simulink model "StateMessage"  (R2024a)
settings: Solver=FixedStepAuto  StartTime=0.0  StopTime=0  FixedStep=0.01  RelTol=1e-3  EnableMultiTasking=on
libraries: MESSIN_Library x3
settings Model: Creator=damerius  LastModifiedBy=Scythe
settings SolverCC: ConcurrentTasks=on  AlgebraicLoopSolver=TrustRegion  PositivePriorityOrder=on
settings DataIOCC: SaveOutput=off  SignalLogging=off  DSMLogging=off  SaveTime=off  ReturnWorkspaceOutputs=off
settings OptimizationCC: DefaultParameterBehavior=Inlined  ReuseModelBlockBuffer=off  ZeroExternalMemoryAtStartup=off  ZeroInternalMemoryAtStartup=off  SimCompilerOptimization=on
settings DebuggingCC: UnconnectedInputMsg=warning  UnconnectedOutputMsg=warning  UnconnectedLineMsg=warning
settings HardwareCC: ProdBitPerLong=64  ProdHWDeviceType=Intel->x86-64 (Linux 64)
settings ModelReferenceCC: EnableRefExpFcnMdlSchedulingChecks=on
settings SFSimCC: SimParseCustomCode=off  SimGenImportedTypeDefs=on  SimTargetLang=C++
settings RTWCC: GenCodeOnly=on  PackageGeneratedCodeAndArtifacts=on  PackageName=PackNGo  RTWVerbose=off  BuildConfiguration=Faster Runs  TargetLang=C++  GPUComputeCapability=3.5  DLArmComputeVersion=19.05
settings CodeAppCC: ForceParamTrailComments=on  MaxIdLength=95  MATLABSourceComments=on  UseSimReservedNames=on
settings GRTTargetCC: TargetLangStandard=C++11 (ISO)  GenerateFullHeader=off  MatFileLogging=off  CodeInterfacePackaging=C++ class

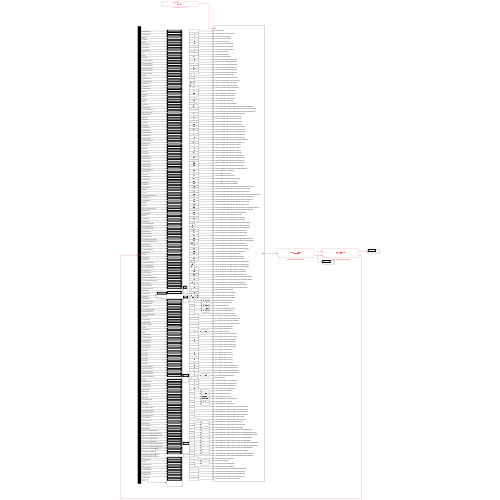
[thumbnail: Simulink's stored preview of the top-level diagram]
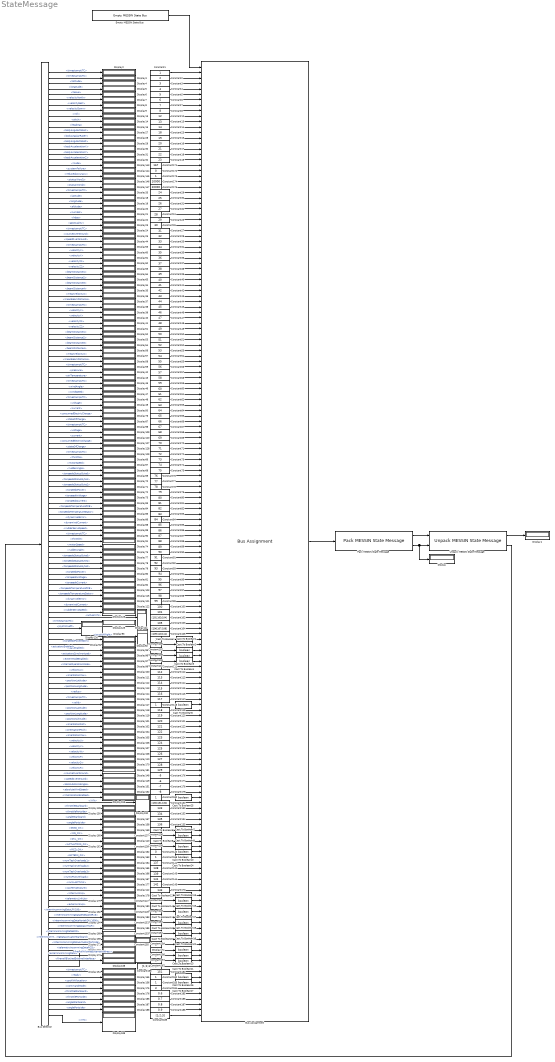
== system StateMessage ==
  Bus Assignment : BusAssignment  AssignedSignals=timestampUTC,sensor.insLFK100.timestampUTC,sensor.insLFK100.latitude,sensor.insLFK100.longitude,sensor.insLFK100.heave,sensor.insLFK100.velocityNorth,sensor.insLFK100.velocityEast,sensor.insLFK100.velocityDown,sensor.insLFK100.roll,sensor.insLFK100.pitch,sensor.insLFK100.heading,sensor.insLFK100.bodyAngularRateX,sensor.insLFK100.bodyAngularRateY,sensor.insLFK100.bodyAngularRateZ,sensor.insLFK100.bodyAccelerationX,sensor.insLFK100.bodyAccelerationY,sensor.insLFK100.bodyAccelerationZ,sensor.insLFK100.details.mode,sensor.insLFK100.details.systemFailure,sensor.insLFK100.details.reducedAccuracy,sensor.insLFK100.details.statusWord1,sensor.insLFK100.details.statusWord2,sensor.gnssAsteRx3.gnss.timestampUTC,sensor.gnssAsteRx3.gnss.latitude,sensor.gnssAsteRx3.gnss.longitude,sensor.gnssAsteRx3.gnss.altitude,sensor.gnssAsteRx3.gnss.numSat,sensor.gnssAsteRx3.gnss.hdop,sensor.gnssAsteRx3.gnss.gpsQuality,sensor.gnssAsteRx3.courseAndSpeedOverGround.timestampUTC,sensor.gnssAsteRx3.courseAndSpeedOverGround.courseOverGround,sensor.gnssAsteRx3.courseAndSpeedOverGround.speedOverGround,sensor.nortekDVL1000.bottomTrack.timestampUTC,sensor.nortekDVL1000.bottomTrack.velocityX,sensor.nortekDVL1000.bottomTrack.velocityY,sensor.nortekDVL1000.bottomTrack.velocityZ1,sensor.nortekDVL1000.bottomTrack.velocityZ2,sensor.nortekDVL1000.bottomTrack.beamDistance1,sensor.nortekDVL1000.bottomTrack.beamDistance2,sensor.nortekDVL1000.bottomTrack.beamDistance3,sensor.nortekDVL1000.bottomTrack.beamDistance4,sensor.nortekDVL1000.bottomTrack.meanVelocityZ,sensor.nortekDVL1000.bottomTrack.meanBeamDistance,sensor.nortekDVL1000.waterTrack.timestampUTC,sensor.nortekDVL1000.waterTrack.velocityX,sensor.nortekDVL1000.waterTrack.velocityY,sensor.nortekDVL1000.waterTrack.velocityZ1,sensor.nortekDVL1000.waterTrack.velocityZ2,sensor.nortekDVL1000.waterTrack.beamDistance1,sensor.nortekDVL1000.waterTrack.beamDistance2,sensor.nortekDVL1000.waterTrack.beamDistance3,sensor.nortekDVL1000.waterTrack.beamDistance4,sensor.nortekDVL1000.waterTrack.meanVelocityZ,sensor.nortekDVL1000.waterTrack.meanBeamDistance,sensor.airMAR.air.timestampUTC,sensor.airMAR.air.pressure,sensor.airMAR.air.airTemperature,sensor.airMAR.relativeWind.timestampUTC,sensor.airMAR.relativeWind.windAngle,sensor.airMAR.relativeWind.windSpeed,sensor.batteryManagementSystem.batteryStarboard.timestampUTC,sensor.batteryManagementSystem.batteryStarboard.voltage,sensor.batteryManagementSystem.batteryStarboard.current,sensor.batteryManagementSystem.batteryStarboard.consumedElectricCharge,sensor.batteryManagementSystem.batteryStarboard.stateOfCharge,sensor.batteryManagementSystem.batteryPortside.timestampUTC,sensor.batteryManagementSystem.batteryPortside.voltage,sensor.batteryManagementSystem.batteryPortside.current,sensor.batteryManagementSystem.batteryPortside.consumedElectricCharge,sensor.batteryManagementSystem.batteryPortside.stateOfCharge,sensor.messinDrive.actuatorStarboard.timestampUTC,sensor.messinDrive.actuatorStarboard.throttle,sensor.messinDrive.actuatorStarboard.motorSpeed,sensor.messinDrive.actuatorStarboard.rudderAngle,sensor.messinDrive.actuatorStarboard.torqeedoStatusByte0,sensor.messinDrive.actuatorStarboard.torqeedoStatusByte1,sensor.messinDrive.actuatorStarboard.torqeedoStatusByte2,sensor.messinDrive.actuatorStarboard.torqeedoPower,sensor.messinDrive.actuatorStarboard.torqeedoVoltage,sensor.messinDrive.actuatorStarboard.torqeedoCurrent,sensor.messinDrive.actuatorStarboard.torqeedoTemperaturePCB,sensor.messinDrive.actuatorStarboard.torqeedoTemperatureStator,sensor.messinDrive.actuatorStarboard.dynamixelError,sensor.messinDrive.actuatorStarboard.dynamixelCurrent,sensor.messinDrive.actuatorStarboard.rudderServoSpeed,sensor.messinDrive.actuatorPortside.timestampUTC,sensor.messinDrive.actuatorPortside.throttle,sensor.messinDrive.actuatorPortside.motorSpeed,sensor.messinDrive.actuatorPortside.rudderAngle,sensor.messinDrive.actuatorPortside.torqeedoStatusByte0,sensor.messinDrive.actuatorPortside.torqeedoStatusByte1,sensor.messinDrive.actuatorPortside.torqeedoStatusByte2,sensor.messinDrive.actuatorPortside.torqeedoPower,sensor.messinDrive.actuatorPortside.torqeedoVoltage,sensor.messinDrive.actuatorPortside.torqeedoCurrent,sensor.messinDrive.actuatorPortside.torqeedoTemperaturePCB,sensor.messinDrive.actuatorPortside.torqeedoTemperatureStator,sensor.messinDrive.actuatorPortside.dynamixelError,sensor.messinDrive.actuatorPortside.dynamixelCurrent,sensor.messinDrive.actuatorPortside.rudderServoSpeed,sensor.messinDrive.actualXYN,remoteControlDevice.timestampUTC,remoteControlDevice.joystickLeft,remoteControlDevice.joystickRight,supervisor.torqeedoPoweredOn,supervisor.actuatorsEnabled,supervisor.lightEnabled,supervisor.actuatorsSynchronized,supervisor.externModeEnabled,supervisor.internalOperationMode,gnc.guidance.surgeHeading.velocityU,gnc.guidance.surgeHeading.orientationYaw,gnc.guidance.stayThere.positionLatitude,gnc.guidance.stayThere.positionLongitude,gnc.guidance.stayThere.radius,gnc.navigation.timestampUTC,gnc.navigation.info.valid,gnc.navigation.state.positionLatitude,gnc.navigation.state.positionLongitude,gnc.navigation.state.positionAltitude,gnc.navigation.state.orientationRoll,gnc.navigation.state.orientationPitch,gnc.navigation.state.orientationYaw,gnc.navigation.state.velocityU,gnc.navigation.state.velocityV,gnc.navigation.state.velocityW,gnc.navigation.state.velocityP,gnc.navigation.state.velocityQ,gnc.navigation.state.velocityR,gnc.navigation.state.courseOverGround,gnc.navigation.state.speedOverGround,gnc.navigation.state.absoluteWindAngle,gnc.navigation.state.absoluteWindSpeed,gnc.control.XNAllocationEnabled,gnc.control.XYN,commandedActuator.throttleStarboard,commandedActuator.throttlePortside,commandedActuator.angleStarboard,commandedActuator.anglePortside,systemDiagnostics.GNSS_OK,systemDiagnostics.INS_OK,systemDiagnostics.DVL_OK,systemDiagnostics.ACTUATORS_OK,systemDiagnostics.RCD_OK,systemDiagnostics.EXTERN_OK,systemDiagnostics.details.hardware.numTaskOverloads1,systemDiagnostics.details.hardware.numTaskOverloads2,systemDiagnostics.details.hardware.numTaskOverloads3,systemDiagnostics.details.hardware.numCPUOverloads,systemDiagnostics.details.hardware.numLostTicks,systemDiagnostics.details.hardware.cpuTemperature,systemDiagnostics.details.network.internLinkUp,systemDiagnostics.details.network.telemetryLinkUp,systemDiagnostics.details.network.externLinkUp,systemDiagnostics.details.network.internIncommingDataLFK100,systemDiagnostics.details.network.internIncommingDataGNSSAsteRx3,systemDiagnostics.details.network.internIncommingDataNortekDVL1000,systemDiagnostics.details.network.internIncommingDataAirMAR,systemDiagnostics.details.network.internIncommingDataBMS,systemDiagnostics.details.network.internIncommingDataActuatorStarboard,systemDiagnostics.details.network.internIncommingDataActuatorPortside,systemDiagnostics.details.network.telemetryIncommingDataRCD,systemDiagnostics.details.network.externIncommingData,systemDiagnostics.details.network.firewallBlockedExternalInterface,systemDiagnostics.details.network.firewallAllowedExternalAddress,externCommand.timestampUTC,externCommand.ready,externCommand.useXNAllocation,externCommand.commandMode,externCommand.actuatorCommand.throttleStarboard,externCommand.actuatorCommand.throttlePortside,externCommand.actuatorCommand.angleStarboard,externCommand.actuatorCommand.anglePortside,externCommand.allocationCommand.XYN
  Bus Selector : BusSelector  OutputSignals=timestampUTC,sensor.insLFK100.timestampUTC,sensor.insLFK100.latitude,sensor.insLFK100.longitude,sensor.insLFK100.heave,sensor.insLFK100.velocityNorth,sensor.insLFK100.velocityEast,sensor.insLFK100.velocityDown,sensor.insLFK100.roll,sensor.insLFK100.pitch,sensor.insLFK100.heading,sensor.insLFK100.bodyAngularRateX,sensor.insLFK100.bodyAngularRateY,sensor.insLFK100.bodyAngularRateZ,sensor.insLFK100.bodyAccelerationX,sensor.insLFK100.bodyAccelerationY,sensor.insLFK100.bodyAccelerationZ,sensor.insLFK100.details.mode,sensor.insLFK100.details.systemFailure,sensor.insLFK100.details.reducedAccuracy,sensor.insLFK100.details.statusWord1,sensor.insLFK100.details.statusWord2,sensor.gnssAsteRx3.gnss.timestampUTC,sensor.gnssAsteRx3.gnss.latitude,sensor.gnssAsteRx3.gnss.longitude,sensor.gnssAsteRx3.gnss.altitude,sensor.gnssAsteRx3.gnss.numSat,sensor.gnssAsteRx3.gnss.hdop,sensor.gnssAsteRx3.gnss.gpsQuality,sensor.gnssAsteRx3.courseAndSpeedOverGround.timestampUTC,sensor.gnssAsteRx3.courseAndSpeedOverGround.courseOverGround,sensor.gnssAsteRx3.courseAndSpeedOverGround.speedOverGround,sensor.nortekDVL1000.bottomTrack.timestampUTC,sensor.nortekDVL1000.bottomTrack.velocityX,sensor.nortekDVL1000.bottomTrack.velocityY,sensor.nortekDVL1000.bottomTrack.velocityZ1,sensor.nortekDVL1000.bottomTrack.velocityZ2,sensor.nortekDVL1000.bottomTrack.beamDistance1,sensor.nortekDVL1000.bottomTrack.beamDistance2,sensor.nortekDVL1000.bottomTrack.beamDistance3,sensor.nortekDVL1000.bottomTrack.beamDistance4,sensor.nortekDVL1000.bottomTrack.meanVelocityZ,sensor.nortekDVL1000.bottomTrack.meanBeamDistance,sensor.nortekDVL1000.waterTrack.timestampUTC,sensor.nortekDVL1000.waterTrack.velocityX,sensor.nortekDVL1000.waterTrack.velocityY,sensor.nortekDVL1000.waterTrack.velocityZ1,sensor.nortekDVL1000.waterTrack.velocityZ2,sensor.nortekDVL1000.waterTrack.beamDistance1,sensor.nortekDVL1000.waterTrack.beamDistance2,sensor.nortekDVL1000.waterTrack.beamDistance3,sensor.nortekDVL1000.waterTrack.beamDistance4,sensor.nortekDVL1000.waterTrack.meanVelocityZ,sensor.nortekDVL1000.waterTrack.meanBeamDistance,sensor.airMAR.air.timestampUTC,sensor.airMAR.air.pressure,sensor.airMAR.air.airTemperature,sensor.airMAR.relativeWind.timestampUTC,sensor.airMAR.relativeWind.windAngle,sensor.airMAR.relativeWind.windSpeed,sensor.batteryManagementSystem.batteryStarboard.timestampUTC,sensor.batteryManagementSystem.batteryStarboard.voltage,sensor.batteryManagementSystem.batteryStarboard.current,sensor.batteryManagementSystem.batteryStarboard.consumedElectricCharge,sensor.batteryManagementSystem.batteryStarboard.stateOfCharge,sensor.batteryManagementSystem.batteryPortside.timestampUTC,sensor.batteryManagementSystem.batteryPortside.voltage,sensor.batteryManagementSystem.batteryPortside.current,sensor.batteryManagementSystem.batteryPortside.consumedElectricCharge,sensor.batteryManagementSystem.batteryPortside.stateOfCharge,sensor.messinDrive.actuatorStarboard.timestampUTC,sensor.messinDrive.actuatorStarboard.throttle,sensor.messinDrive.actuatorStarboard.motorSpeed,sensor.messinDrive.actuatorStarboard.rudderAngle,sensor.messinDrive.actuatorStarboard.torqeedoStatusByte0,sensor.messinDrive.actuatorStarboard.torqeedoStatusByte1,sensor.messinDrive.actuatorStarboard.torqeedoStatusByte2,sensor.messinDrive.actuatorStarboard.torqeedoPower,sensor.messinDrive.actuatorStarboard.torqeedoVoltage,sensor.messinDrive.actuatorStarboard.torqeedoCurrent,sensor.messinDrive.actuatorStarboard.torqeedoTemperaturePCB,sensor.messinDrive.actuatorStarboard.torqeedoTemperatureStator,sensor.messinDrive.actuatorStarboard.dynamixelError,sensor.messinDrive.actuatorStarboard.dynamixelCurrent,sensor.messinDrive.actuatorStarboard.rudderServoSpeed,sensor.messinDrive.actuatorPortside.timestampUTC,sensor.messinDrive.actuatorPortside.throttle,sensor.messinDrive.actuatorPortside.motorSpeed,sensor.messinDrive.actuatorPortside.rudderAngle,sensor.messinDrive.actuatorPortside.torqeedoStatusByte0,sensor.messinDrive.actuatorPortside.torqeedoStatusByte1,sensor.messinDrive.actuatorPortside.torqeedoStatusByte2,sensor.messinDrive.actuatorPortside.torqeedoPower,sensor.messinDrive.actuatorPortside.torqeedoVoltage,sensor.messinDrive.actuatorPortside.torqeedoCurrent,sensor.messinDrive.actuatorPortside.torqeedoTemperaturePCB,sensor.messinDrive.actuatorPortside.torqeedoTemperatureStator,sensor.messinDrive.actuatorPortside.dynamixelError,sensor.messinDrive.actuatorPortside.dynamixelCurrent,sensor.messinDrive.actuatorPortside.rudderServoSpeed,sensor.messinDrive.actualXYN,remoteControlDevice.timestampUTC,remoteControlDevice.joystickLeft,remoteControlDevice.joystickRight,supervisor.torqeedoPoweredOn,supervisor.actuatorsEnabled,supervisor.lightEnabled,supervisor.actuatorsSynchronized,supervisor.externModeEnabled,supervisor.internalOperationMode,gnc.guidance.surgeHeading.velocityU,gnc.guidance.surgeHeading.orientationYaw,gnc.guidance.stayThere.positionLatitude,gnc.guidance.stayThere.positionLongitude,gnc.guidance.stayThere.radius,gnc.navigation.timestampUTC,gnc.navigation.info.valid,gnc.navigation.state.positionLatitude,gnc.navigation.state.positionLongitude,gnc.navigation.state.positionAltitude,gnc.navigation.state.orientationRoll,gnc.navigation.state.orientationPitch,gnc.navigation.state.orientationYaw,gnc.navigation.state.velocityU,gnc.navigation.state.velocityV,gnc.navigation.state.velocityW,gnc.navigation.state.velocityP,gnc.navigation.state.velocityQ,gnc.navigation.state.velocityR,gnc.navigation.state.courseOverGround,gnc.navigation.state.speedOverGround,gnc.navigation.state.absoluteWindAngle,gnc.navigation.state.absoluteWindSpeed,gnc.control.XNAllocationEnabled,gnc.control.XYN,commandedActuator.throttleStarboard,commandedActuator.throttlePortside,commandedActuator.angleStarboard,commandedActuator.anglePortside,systemDiagnostics.GNSS_OK,systemDiagnostics.INS_OK,systemDiagnostics.DVL_OK,systemDiagnostics.ACTUATORS_OK,systemDiagnostics.RCD_OK,systemDiagnostics.EXTERN_OK,systemDiagnostics.details.hardware.numTaskOverloads1,systemDiagnostics.details.hardware.numTaskOverloads2,systemDiagnostics.details.hardware.numTaskOverloads3,systemDiagnostics.details.hardware.numCPUOverloads,systemDiagnostics.details.hardware.numLostTicks,systemDiagnostics.details.hardware.cpuTemperature,systemDiagnostics.details.network.internLinkUp,systemDiagnostics.details.network.telemetryLinkUp,systemDiagnostics.details.network.externLinkUp,systemDiagnostics.details.network.internIncommingDataLFK100,systemDiagnostics.details.network.internIncommingDataGNSSAsteRx3,systemDiagnostics.details.network.internIncommingDataNortekDVL1000,systemDiagnostics.details.network.internIncommingDataAirMAR,systemDiagnostics.details.network.internIncommingDataBMS,systemDiagnostics.details.network.internIncommingDataActuatorStarboard,systemDiagnostics.details.network.internIncommingDataActuatorPortside,systemDiagnostics.details.network.telemetryIncommingDataRCD,systemDiagnostics.details.network.externIncommingData,systemDiagnostics.details.network.firewallBlockedExternalInterface,systemDiagnostics.details.network.firewallAllowedExternalAddress,externCommand.timestampUTC,externCommand.ready,externCommand.useXNAllocation,externCommand.commandMode,externCommand.actuatorCommand.throttleStarboard,externCommand.actuatorCommand.throttlePortside,externCommand.actuatorCommand.angleStarboard,externCommand.actuatorCommand.anglePortside,externCommand.allocationCommand.XYN
  Cast To Boolean{,1..27} (28 alike) : DataTypeConversion  OutDataTypeStr=boolean  SaturateOnIntegerOverflow=off  RndMeth=Floor
  Constant1 : Constant  OutDataTypeStr=double
  Constant100 : Constant  Value=100  OutDataTypeStr=double
  Constant101 : Constant  Value=101  OutDataTypeStr=double
  Constant102 : Constant  Value=[102;103;104]  OutDataTypeStr=double
  Constant103 : Constant  Value=105  OutDataTypeStr=double
  Constant104 : Constant  Value=[106;107;108]  OutDataTypeStr=double
  Constant105 : Constant  Value=[109;110;111]  OutDataTypeStr=double
  Constant{106,108,110..111,118,136,138..139,146..147,149..150,152..153,155..156,168,180,182..183} (20 alike) : Constant  OutDataTypeStr=uint8
  Constant{107,109,137,140,148,151,154,157,167} (9 alike) : Constant  Value=0  OutDataTypeStr=uint8
  Constant112 : Constant  Value=112  OutDataTypeStr=double
  Constant113 : Constant  Value=113  OutDataTypeStr=double
  Constant114 : Constant  Value=114  OutDataTypeStr=double
  Constant115 : Constant  Value=115  OutDataTypeStr=double
  Constant116 : Constant  Value=116  OutDataTypeStr=double
  Constant117 : Constant  Value=117  OutDataTypeStr=double
  Constant119 : Constant  Value=118  OutDataTypeStr=double
  Constant12 : Constant  Value=12  OutDataTypeStr=double
  Constant120 : Constant  Value=119  OutDataTypeStr=double
  Constant121 : Constant  Value=120  OutDataTypeStr=double
  Constant122 : Constant  Value=121  OutDataTypeStr=double
  Constant123 : Constant  Value=122  OutDataTypeStr=double
  Constant124 : Constant  Value=123  OutDataTypeStr=double
  Constant125 : Constant  Value=124  OutDataTypeStr=double
  Constant126 : Constant  Value=125  OutDataTypeStr=double
  Constant127 : Constant  Value=126  OutDataTypeStr=double
  Constant128 : Constant  Value=127  OutDataTypeStr=double
  Constant129 : Constant  Value=128  OutDataTypeStr=double
  Constant13 : Constant  Value=13  OutDataTypeStr=double
  Constant130 : Constant  Value=129  OutDataTypeStr=double
  Constant131 : Constant  Value=[130;131;132]  OutDataTypeStr=double
  Constant132 : Constant  Value=133  OutDataTypeStr=double
  Constant133 : Constant  Value=134  OutDataTypeStr=double
  Constant134 : Constant  Value=135  OutDataTypeStr=double
  Constant135 : Constant  Value=136  OutDataTypeStr=double
  Constant14 : Constant  Value=14  OutDataTypeStr=double
  Constant141 : Constant  Value=137  OutDataTypeStr=uint32
  Constant142 : Constant  Value=138  OutDataTypeStr=uint32
  Constant143 : Constant  Value=139  OutDataTypeStr=uint32
  Constant144 : Constant  Value=141  OutDataTypeStr=uint32
  Constant145 : Constant  Value=142  OutDataTypeStr=uint32
  Constant15 : Constant  Value=19  OutDataTypeStr=double
  Constant158 : Constant  Value=[1;2;3;4;5]  OutDataTypeStr=uint16
  Constant16 : Constant  Value=20  OutDataTypeStr=double
  Constant17 : Constant  Value=21  OutDataTypeStr=double
  Constant170 : Constant  Value=143  OutDataTypeStr=double
  Constant171 : Constant  Value=167  OutDataTypeStr=uint8
  Constant172 : Constant  Value=0  OutDataTypeStr=boolean
  Constant173 : Constant  OutDataTypeStr=boolean
  Constant174 : Constant  Value=10000  OutDataTypeStr=uint16
  Constant175 : Constant  Value=20000  OutDataTypeStr=uint16
  Constant176 : Constant  Value=-5  OutDataTypeStr=double
  Constant177 : Constant  Value=-6  OutDataTypeStr=double
  Constant178 : Constant  Value=-7  OutDataTypeStr=double
  Constant179 : Constant  Value=-8  OutDataTypeStr=double
  Constant18 : Constant  Value=22  OutDataTypeStr=double
  Constant181 : Constant  Value=151  OutDataTypeStr=double
  Constant184 : Constant  Value=3  OutDataTypeStr=uint8
  Constant185 : Constant  Value=0.6  OutDataTypeStr=double
  Constant186 : Constant  Value=0.7  OutDataTypeStr=double
  Constant187 : Constant  Value=0.8  OutDataTypeStr=double
  Constant188 : Constant  Value=0.9  OutDataTypeStr=double
  Constant189 : Constant  Value=[1;2;3]  OutDataTypeStr=double
  Constant19 : Constant  Value=23  OutDataTypeStr=double
  Constant2 : Constant  Value=2  OutDataTypeStr=double
  Constant23 : Constant  Value=18  OutDataTypeStr=double
  Constant24 : Constant  Value=28  OutDataTypeStr=uint8
  Constant25 : Constant  Value=29  OutDataTypeStr=double
  Constant26 : Constant  Value=30  OutDataTypeStr=uint8
  Constant27 : Constant  Value=31  OutDataTypeStr=double
  Constant28 : Constant  Value=32  OutDataTypeStr=double
  Constant29 : Constant  Value=24  OutDataTypeStr=double
  Constant3 : Constant  Value=3  OutDataTypeStr=double
  Constant30 : Constant  Value=25  OutDataTypeStr=double
  Constant31 : Constant  Value=26  OutDataTypeStr=double
  Constant32 : Constant  Value=27  OutDataTypeStr=double
  Constant33 : Constant  Value=33  OutDataTypeStr=double
  Constant34 : Constant  Value=34  OutDataTypeStr=double
  Constant35 : Constant  Value=35  OutDataTypeStr=double
  Constant36 : Constant  Value=36  OutDataTypeStr=double
  Constant37 : Constant  Value=37  OutDataTypeStr=double
  Constant38 : Constant  Value=38  OutDataTypeStr=double
  Constant39 : Constant  Value=39  OutDataTypeStr=double
  Constant4 : Constant  Value=4  OutDataTypeStr=double
  Constant40 : Constant  Value=40  OutDataTypeStr=double
  Constant41 : Constant  Value=41  OutDataTypeStr=double
  Constant42 : Constant  Value=42  OutDataTypeStr=double
  Constant43 : Constant  Value=43  OutDataTypeStr=double
  Constant44 : Constant  Value=44  OutDataTypeStr=double
  Constant45 : Constant  Value=45  OutDataTypeStr=double
  Constant46 : Constant  Value=46  OutDataTypeStr=double
  Constant47 : Constant  Value=47  OutDataTypeStr=double
  Constant48 : Constant  Value=48  OutDataTypeStr=double
  Constant49 : Constant  Value=49  OutDataTypeStr=double
  Constant5 : Constant  Value=5  OutDataTypeStr=double
  Constant50 : Constant  Value=50  OutDataTypeStr=double
  Constant51 : Constant  Value=51  OutDataTypeStr=double
  Constant52 : Constant  Value=52  OutDataTypeStr=double
  Constant53 : Constant  Value=53  OutDataTypeStr=double
  Constant54 : Constant  Value=54  OutDataTypeStr=double
  Constant55 : Constant  Value=55  OutDataTypeStr=double
  Constant56 : Constant  Value=56  OutDataTypeStr=double
  Constant57 : Constant  Value=57  OutDataTypeStr=double
  Constant58 : Constant  Value=58  OutDataTypeStr=double
  Constant59 : Constant  Value=59  OutDataTypeStr=double
  Constant6 : Constant  Value=6  OutDataTypeStr=double
  Constant60 : Constant  Value=60  OutDataTypeStr=double
  Constant61 : Constant  Value=61  OutDataTypeStr=double
  Constant62 : Constant  Value=62  OutDataTypeStr=double
  Constant63 : Constant  Value=63  OutDataTypeStr=double
  Constant64 : Constant  Value=64  OutDataTypeStr=double
  Constant65 : Constant  Value=65  OutDataTypeStr=double
  Constant66 : Constant  Value=66  OutDataTypeStr=double
  Constant67 : Constant  Value=67  OutDataTypeStr=double
  Constant68 : Constant  Value=68  OutDataTypeStr=double
  Constant69 : Constant  Value=69  OutDataTypeStr=double
  Constant7 : Constant  Value=7  OutDataTypeStr=double
  Constant70 : Constant  Value=70  OutDataTypeStr=double
  Constant71 : Constant  Value=71  OutDataTypeStr=double
  Constant72 : Constant  Value=72  OutDataTypeStr=double
  Constant73 : Constant  Value=73  OutDataTypeStr=double
  Constant74 : Constant  Value=74  OutDataTypeStr=double
  Constant75 : Constant  Value=75  OutDataTypeStr=double
  Constant76 : Constant  Value=76  OutDataTypeStr=uint8
  Constant77 : Constant  Value=77  OutDataTypeStr=uint8
  Constant78 : Constant  Value=78  OutDataTypeStr=uint8
  Constant79 : Constant  Value=79  OutDataTypeStr=double
  Constant8 : Constant  Value=8  OutDataTypeStr=double
  Constant80 : Constant  Value=80  OutDataTypeStr=double
  Constant81 : Constant  Value=81  OutDataTypeStr=double
  Constant82 : Constant  Value=82  OutDataTypeStr=double
  Constant83 : Constant  Value=83  OutDataTypeStr=double
  Constant84 : Constant  Value=84  OutDataTypeStr=uint8
  Constant85 : Constant  Value=85  OutDataTypeStr=double
  Constant86 : Constant  Value=86  OutDataTypeStr=double
  Constant87 : Constant  Value=87  OutDataTypeStr=double
  Constant88 : Constant  Value=88  OutDataTypeStr=double
  Constant89 : Constant  Value=89  OutDataTypeStr=double
  Constant90 : Constant  Value=90  OutDataTypeStr=double
  Constant91 : Constant  Value=91  OutDataTypeStr=uint8
  Constant92 : Constant  Value=92  OutDataTypeStr=uint8
  Constant93 : Constant  Value=93  OutDataTypeStr=uint8
  Constant94 : Constant  Value=94  OutDataTypeStr=double
  Constant95 : Constant  Value=95  OutDataTypeStr=double
  Constant96 : Constant  Value=96  OutDataTypeStr=double
  Constant97 : Constant  Value=97  OutDataTypeStr=double
  Constant98 : Constant  Value=98  OutDataTypeStr=double
  Constant99 : Constant  Value=99  OutDataTypeStr=uint8
  Display{,1..9,13..15,18..25,27..129,138..140,142..189,192} (176 alike) : Display
  Empty MESSIN State Bus : MESSIN_Library/State Message/Empty MESSIN State Bus
      settings: SourceProductName=MESSIN - Interface Library
  Pack MESSIN State Message : MESSIN_Library/State Message/Pack MESSIN State Message
      settings: SourceProductName=MESSIN - Interface Library
  Unpack MESSIN State Message : MESSIN_Library/State Message/Unpack MESSIN State Message
      settings: SourceProductName=MESSIN - Interface Library
  wires:
  Bus Selector/174 -> Display189/1  "<XYN>"
  Bus Selector/170 -> Display176/1  "<throttleStarboard>"
  Bus Selector/171 -> Display186/1  "<throttlePortside>"
  Bus Selector/173 -> Display188/1  "<anglePortside>"
  Bus Selector/172 -> Display187/1  "<angleStarboard>"
  Bus Selector/168 -> Display156/1  "<useXNAllocation>"
  Bus Selector/169 -> Display175/1  "<commandMode>"
  Bus Selector/167 -> Display155/1  "<ready>"
  Bus Selector/166 -> Display154/1  "<timestampUTC>"
  Constant189/1 -> Bus Assignment/175
  Constant188/1 -> Bus Assignment/174
  Constant187/1 -> Bus Assignment/173
  Constant186/1 -> Bus Assignment/172
  Constant185/1 -> Bus Assignment/171
  Constant184/1 -> Bus Assignment/170
  Cast To Boolean27/1 -> Bus Assignment/169
  Cast To Boolean26/1 -> Bus Assignment/168
  Constant182/1 -> Cast To Boolean26/1
  Constant183/1 -> Cast To Boolean27/1
  Constant181/1 -> Bus Assignment/167
  Cast To Boolean25/1 -> Bus Assignment/135
  Constant180/1 -> Cast To Boolean25/1
  Bus Selector/134 -> Display153/1  "<XNAllocationEnabled>"
  Bus Selector/133 -> Display152/1  "<absoluteWindSpeed>"
  Bus Selector/132 -> Display151/1  "<absoluteWindAngle>"
  Bus Selector/131 -> Display149/1  "<speedOverGround>"
  Bus Selector/130 -> Display148/1  "<courseOverGround>"
  Constant179/1 -> Bus Assignment/134
  Constant178/1 -> Bus Assignment/133
  Constant177/1 -> Bus Assignment/132
  Constant176/1 -> Bus Assignment/131
  Bus Selector/22 -> Display147/1  "<statusWord2>"
  Bus Selector/21 -> Display146/1  "<statusWord1>"
  Bus Selector/20 -> Display145/1  "<reducedAccuracy>"
  Bus Selector/19 -> Display144/1  "<systemFailure>"
  Bus Selector/18 -> Display143/1  "<mode>"
  Constant175/1 -> Bus Assignment/23
  Constant174/1 -> Bus Assignment/22
  Constant173/1 -> Bus Assignment/21
  Constant172/1 -> Bus Assignment/20
  Constant171/1 -> Bus Assignment/19
  Constant170/1 -> Bus Assignment/152
  Bus Selector/151 -> Display142/1  "<cpuTemperature>"
  Bus Selector/145 -> Display163/1  "<EXTERN_OK>"
  Bus Selector/144 -> Display162/1  "<RCD_OK>"
  Bus Selector/143 -> Display161/1  "<ACTUATORS_OK>"
  Bus Selector/142 -> Display140/1  "<DVL_OK>"
  Bus Selector/141 -> Display160/1  "<INS_OK>"
  Bus Selector/140 -> Display159/1  "<GNSS_OK>"
  Cast To Boolean6/1 -> Bus Assignment/141
  Cast To Boolean7/1 -> Bus Assignment/142
  Cast To Boolean8/1 -> Bus Assignment/143
  Cast To Boolean9/1 -> Bus Assignment/144
  Cast To Boolean10/1 -> Bus Assignment/145
  Cast To Boolean24/1 -> Bus Assignment/146
  Constant168/1 -> Cast To Boolean24/1
  Bus Selector/164 -> Display138/1  "<firewallBlockedExternalInterface>"
  Bus Selector/163 -> Display173/1  "<externIncommingData>"
  Bus Selector/162 -> Display172/1  "<telemetryIncommingDataRCD>"
  Bus Selector/161 -> Display171/1  "<internIncommingDataActuatorPortside>"
  Bus Selector/160 -> Display169/1  "<internIncommingDataActuatorStarboard>"
  Bus Selector/159 -> Display168/1  "<internIncommingDataBMS>"
  Bus Selector/158 -> Display185/1  "<internIncommingDataAirMAR>"
  Bus Selector/157 -> Display184/1  "<internIncommingDataNortekDVL1000>"
  Bus Selector/156 -> Display183/1  "<internIncommingDataGNSSAsteRx3>"
  Bus Selector/155 -> Display182/1  "<internIncommingDataLFK100>"
  Bus Selector/154 -> Display180/1  "<externLinkUp>"
  Bus Selector/153 -> Display179/1  "<telemetryLinkUp>"
  Bus Selector/165 -> Display174/1  "<firewallAllowedExternalAddress>"
  Cast To Boolean21/1 -> Bus Assignment/165
  Cast To Boolean23/1 -> Bus Assignment/164
  Cast To Boolean22/1 -> Bus Assignment/163
  Cast To Boolean16/1 -> Bus Assignment/162
  Cast To Boolean20/1 -> Bus Assignment/161
  Cast To Boolean19/1 -> Bus Assignment/160
  Cast To Boolean18/1 -> Bus Assignment/159
  Cast To Boolean17/1 -> Bus Assignment/158
  Cast To Boolean11/1 -> Bus Assignment/157
  Cast To Boolean15/1 -> Bus Assignment/156
  Cast To Boolean14/1 -> Bus Assignment/155
  Cast To Boolean13/1 -> Bus Assignment/154
  Constant167/1 -> Cast To Boolean21/1
  Bus Assignment/1 -> Pack MESSIN State Message/1
  Bus Selector/4 -> Display5/1  "<longitude>"
  Constant131/1 -> Bus Assignment/136
  Constant157/1 -> Cast To Boolean23/1
  Bus Selector/7 -> Display8/1  "<velocityEast>"
  Constant149/1 -> Cast To Boolean15/1
  Constant101/1 -> Bus Assignment/101
  Constant135/1 -> Bus Assignment/140
  Constant35/1 -> Bus Assignment/35
  Constant29/1 -> Bus Assignment/24
  Constant112/1 -> Bus Assignment/112
  Constant110/1 -> Cast To Boolean4/1
  Constant107/1 -> Cast To Boolean1/1
  Constant72/1 -> Bus Assignment/72
  Constant77/1 -> Bus Assignment/77
  Constant83/1 -> Bus Assignment/83
  Constant63/1 -> Bus Assignment/63
  Constant84/1 -> Bus Assignment/84
  Constant97/1 -> Bus Assignment/97
  Constant55/1 -> Bus Assignment/55
  Constant44/1 -> Bus Assignment/44
  Constant45/1 -> Bus Assignment/45
  Constant39/1 -> Bus Assignment/39
  Constant61/1 -> Bus Assignment/61
  Cast To Boolean4/1 -> Bus Assignment/110
  Constant62/1 -> Bus Assignment/62
  Constant26/1 -> Bus Assignment/30
  Constant36/1 -> Bus Assignment/36
  Constant25/1 -> Bus Assignment/29
  Constant34/1 -> Bus Assignment/34
  Constant105/1 -> Bus Assignment/105
  Constant30/1 -> Bus Assignment/25
  Constant5/1 -> Bus Assignment/6
  Constant56/1 -> Bus Assignment/56
  Constant1/1 -> Bus Assignment/2
  Constant16/1 -> Bus Assignment/15
  Constant7/1 -> Bus Assignment/8
  Constant3/1 -> Bus Assignment/4
  Constant15/1 -> Bus Assignment/14
  Constant156/1 -> Cast To Boolean22/1
  Constant27/1 -> Bus Assignment/31
  Bus Selector/66 -> Display98/1  "<timestampUTC>"
  Constant24/1 -> Bus Assignment/28
  Pack MESSIN State Message/1 -> Unpack MESSIN State Message/1
  Bus Selector/137 -> Display150/1  "<throttlePortside>"
  Bus Selector/146 -> Display164/1  "<numTaskOverloads1>"
  Constant95/1 -> Bus Assignment/95
  Bus Selector/49 -> Display52/1  "<beamDistance1>"
  Bus Selector/152 -> Display178/1  "<internLinkUp>"
  Bus Selector/24 -> Display18/1  "<latitude>"
  Bus Selector/30 -> Display24/1  "<timestampUTC>"
  Bus Selector/113 -> Display112/1  "<positionLatitude>"
  Constant65/1 -> Bus Assignment/65
  Bus Selector/147 -> Display165/1  "<numTaskOverloads2>"
  Constant49/1 -> Bus Assignment/49
  Bus Selector/87 -> Display91/1  "<throttle>"
  Bus Selector/75 -> Display69/1  "<torqeedoStatusByte0>"
  Constant41/1 -> Bus Assignment/41
  Constant42/1 -> Bus Assignment/42
  Constant109/1 -> Cast To Boolean3/1
  Bus Selector/103 -> Display126/1  "<joystickLeft>"
  Constant8/1 -> Bus Assignment/9
  Constant33/1 -> Bus Assignment/33
  Bus Selector/149 -> Display167/1  "<numCPUOverloads>"
  Constant12/1 -> Bus Assignment/10
  Constant116/1 -> Bus Assignment/116
  Bus Selector/129 -> Display181/1  "<velocityR>"
  Bus Selector/48 -> Display51/1  "<velocityZ2>"
  Constant122/1 -> Bus Assignment/122
  Constant19/1 -> Bus Assignment/18
  Bus Selector/138 -> Display157/1  "<angleStarboard>"
  Constant148/1 -> Cast To Boolean14/1
  Bus Selector/136 -> Display139/1  "<throttleStarboard>"
  Constant51/1 -> Bus Assignment/51
  Bus Selector/120 -> Display101/1  "<positionAltitude>"
  Constant68/1 -> Bus Assignment/68
  Bus Selector/121 -> Display102/1  "<orientationRoll>"
  Cast To Boolean12/1 -> Bus Assignment/153
  Bus Selector/105 -> Display93/1  "<torqeedoPoweredOn>"
  Bus Selector/123 -> Display105/1  "<orientationYaw>"
  Bus Selector/38 -> Display64/1  "<beamDistance1>"
  Bus Selector/119 -> Display119/1  "<positionLongitude>"
  Constant147/1 -> Cast To Boolean13/1
  Constant93/1 -> Bus Assignment/93
  Bus Selector/61 -> Display48/1  "<timestampUTC>"
  Bus Selector/118 -> Display118/1  "<positionLatitude>"
  Bus Selector/64 -> Display76/1  "<consumedElectricCharge>"
  Constant78/1 -> Bus Assignment/78
  Empty MESSIN State Bus/1 -> Bus Assignment/1
  Bus Selector/117 -> Display117/1  "<valid>"
  Cast To Boolean/1 -> Bus Assignment/106
  Bus Selector/70 -> Display128/1  "<stateOfCharge>"
  Constant129/1 -> Bus Assignment/129
  Constant139/1 -> Cast To Boolean9/1
  Bus Selector/5 -> Display6/1  "<heave>"
  Constant6/1 -> Bus Assignment/7
  Bus Selector/128 -> Display170/1  "<velocityQ>"
  Constant86/1 -> Bus Assignment/86
  Constant82/1 -> Bus Assignment/82
  Bus Selector/111 -> Display100/1  "<velocityU>"
  Constant117/1 -> Bus Assignment/117
  Bus Selector/50 -> Display53/1  "<beamDistance2>"
  Constant144/1 -> Bus Assignment/150
  Constant59/1 -> Bus Assignment/59
  Bus Selector/112 -> Display111/1  "<orientationYaw>"
  Constant23/1 -> Bus Assignment/13
  Cast To Boolean3/1 -> Bus Assignment/109
  Bus Selector/100 -> Display123/1  "<rudderServoSpeed>"
  Bus Selector/90 -> Display77/1  "<torqeedoStatusByte0>"
  Bus Selector/104 -> Display92/1  "<joystickRight>"
  Constant87/1 -> Bus Assignment/87
  Constant136/1 -> Cast To Boolean6/1
  Constant130/1 -> Bus Assignment/130
  Constant47/1 -> Bus Assignment/47
  Constant111/1 -> Bus Assignment/111
  Bus Selector/92 -> Display79/1  "<torqeedoStatusByte2>"
  Constant104/1 -> Bus Assignment/104
  Constant81/1 -> Bus Assignment/81
  Bus Selector/72 -> Display66/1  "<throttle>"
  Constant92/1 -> Bus Assignment/92
  Constant53/1 -> Bus Assignment/53
  Constant4/1 -> Bus Assignment/5
  Constant28/1 -> Bus Assignment/32
  Bus Selector/59 -> Display46/1  "<windAngle>"
  Bus Selector/88 -> Display74/1  "<motorSpeed>"
  Bus Selector/116 -> Display116/1  "<timestampUTC>"
  Bus Selector/101 -> Display124/1  "<actualXYN>"
  Cast To Boolean2/1 -> Bus Assignment/108
  Constant52/1 -> Bus Assignment/52
  Constant99/1 -> Bus Assignment/99
  Constant79/1 -> Bus Assignment/79
  Constant91/1 -> Bus Assignment/91
  Bus Selector/11 -> Display15/1  "<heading>"
  Constant43/1 -> Bus Assignment/43
  Bus Selector/13 -> Display28/1  "<bodyAngularRateY>"
  Constant126/1 -> Bus Assignment/126
  Constant96/1 -> Bus Assignment/96
  Bus Selector/44 -> Display38/1  "<timestampUTC>"
  Bus Selector/32 -> Display44/1  "<speedOverGround>"
  Bus Selector/115 -> Display114/1  "<radius>"
  Constant119/1 -> Bus Assignment/119
  Constant133/1 -> Bus Assignment/138
  Bus Selector/31 -> Display25/1  "<courseOverGround>"
  Bus Selector/84 -> Display88/1  "<dynamixelCurrent>"
  Bus Selector/102 -> Display125/1  "<timestampUTC>"
  Bus Selector/77 -> Display71/1  "<torqeedoStatusByte2>"
  Constant114/1 -> Bus Assignment/114
  Bus Selector/79 -> Display73/1  "<torqeedoVoltage>"
  Bus Selector/86 -> Display90/1  "<timestampUTC>"
  Bus Selector/93 -> Display80/1  "<torqeedoPower>"
  Bus Selector/55 -> Display59/1  "<timestampUTC>"
  Bus Selector/135 -> Display192/1  "<XYN>"
  Bus Selector/74 -> Display68/1  "<rudderAngle>"
  Constant40/1 -> Bus Assignment/40
  Bus Selector/29 -> Display23/1  "<gpsQuality>"
  Constant48/1 -> Bus Assignment/48
  Bus Selector/139 -> Display158/1  "<anglePortside>"
  Constant80/1 -> Bus Assignment/80
  Bus Selector/6 -> Display7/1  "<velocityNorth>"
  Bus Selector/12 -> Display27/1  "<bodyAngularRateX>"
  Bus Selector/60 -> Display47/1  "<windSpeed>"
  Bus Selector/94 -> Display81/1  "<torqeedoVoltage>"
  Bus Selector/98 -> Display121/1  "<dynamixelError>"
  Bus Selector/57 -> Display43/1  "<airTemperature>"
  Bus Selector/62 -> Display49/1  "<voltage>"
  Bus Selector/73 -> Display67/1  "<motorSpeed>"
  Unpack MESSIN State Message/2 -> Bus Selector/1
  Bus Selector/91 -> Display78/1  "<torqeedoStatusByte1>"
  Bus Selector/76 -> Display70/1  "<torqeedoStatusByte1>"
  Constant71/1 -> Bus Assignment/71
  Bus Selector/56 -> Display42/1  "<pressure>"
  Bus Selector/47 -> Display41/1  "<velocityZ1>"
  Bus Selector/68 -> Display120/1  "<current>"
  Constant138/1 -> Cast To Boolean8/1
  Constant70/1 -> Bus Assignment/70
  Bus Selector/69 -> Display127/1  "<consumedElectricCharge>"
  Constant140/1 -> Cast To Boolean10/1
  Bus Selector/43 -> Display37/1  "<meanBeamDistance>"
  Bus Selector/71 -> Display129/1  "<timestampUTC>"
  Pack MESSIN State Message/2 -> Unpack MESSIN State Message/2, Display/1
  Cast To Boolean1/1 -> Bus Assignment/107
  Bus Selector/83 -> Display86/1  "<dynamixelError>"
  Constant64/1 -> Bus Assignment/64
  Constant85/1 -> Bus Assignment/85
  Bus Selector/40 -> Display34/1  "<beamDistance3>"
  Bus Selector/99 -> Display122/1  "<dynamixelCurrent>"
  Bus Selector/52 -> Display56/1  "<beamDistance4>"
  Bus Selector/107 -> Display95/1  "<lightEnabled>"
  Bus Selector/63 -> Display50/1  "<current>"
  Bus Selector/37 -> Display63/1  "<velocityZ2>"
  Constant151/1 -> Cast To Boolean17/1
  Bus Selector/97 -> Display115/1  "<torqeedoTemperatureStator>"
  Constant146/1 -> Cast To Boolean12/1
  Bus Selector/89 -> Display75/1  "<rudderAngle>"
  Bus Selector/39 -> Display65/1  "<beamDistance2>"
  Bus Selector/36 -> Display62/1  "<velocityZ1>"
  Bus Selector/33 -> Display55/1  "<timestampUTC>"
  Constant154/1 -> Cast To Boolean20/1
  Bus Selector/3 -> Display4/1  "<latitude>"
  Bus Selector/58 -> Display45/1  "<timestampUTC>"
  Constant38/1 -> Bus Assignment/38
  Constant137/1 -> Cast To Boolean7/1
  Bus Selector/110 -> Display99/1  "<internalOperationMode>"
  Bus Selector/25 -> Display19/1  "<longitude>"
  Bus Selector/65 -> Display87/1  "<stateOfCharge>"
  Bus Selector/16 -> Display31/1  "<bodyAccelerationY>"
  Constant128/1 -> Bus Assignment/128
  Constant142/1 -> Bus Assignment/148
  Constant14/1 -> Bus Assignment/12
  Constant102/1 -> Bus Assignment/102
  Bus Selector/80 -> Display83/1  "<torqeedoCurrent>"
  Bus Selector/122 -> Display104/1  "<orientationPitch>"
  Bus Selector/46 -> Display40/1  "<velocityY>"
  Bus Selector/124 -> Display106/1  "<velocityU>"
  Bus Selector/14 -> Display29/1  "<bodyAngularRateZ>"
  Constant76/1 -> Bus Assignment/76
  Constant94/1 -> Bus Assignment/94
  Constant141/1 -> Bus Assignment/147
  Bus Selector/54 -> Display58/1  "<meanBeamDistance>"
  Bus Selector/17 -> Display32/1  "<bodyAccelerationZ>"
  Constant153/1 -> Cast To Boolean19/1
  Constant98/1 -> Bus Assignment/98
  Bus Selector/108 -> Display96/1  "<actuatorsSynchronized>"
  Constant143/1 -> Bus Assignment/149
  Constant66/1 -> Bus Assignment/66
  Constant125/1 -> Bus Assignment/125
  Constant155/1 -> Cast To Boolean16/1
  Bus Selector/15 -> Display30/1  "<bodyAccelerationX>"
  Constant127/1 -> Bus Assignment/127
  Constant73/1 -> Bus Assignment/73
  Bus Selector/28 -> Display22/1  "<hdop>"
  Bus Selector/78 -> Display72/1  "<torqeedoPower>"
  Constant120/1 -> Bus Assignment/120
  Constant75/1 -> Bus Assignment/75
  Constant124/1 -> Bus Assignment/124
  Bus Selector/10 -> Display14/1  "<pitch>"
  Constant13/1 -> Bus Assignment/11
  Bus Selector/9 -> Display13/1  "<roll>"
  Bus Selector/125 -> Display107/1  "<velocityV>"
  Constant18/1 -> Bus Assignment/17
  Constant74/1 -> Bus Assignment/74
  Bus Selector/41 -> Display35/1  "<beamDistance4>"
  Bus Selector/81 -> Display84/1  "<torqeedoTemperaturePCB>"
  Constant31/1 -> Bus Assignment/26
  Constant2/1 -> Bus Assignment/3
  Constant67/1 -> Bus Assignment/67
  Constant54/1 -> Bus Assignment/54
  Bus Selector/126 -> Display108/1  "<velocityW>"
  Constant158/1 -> Bus Assignment/166
  Constant103/1 -> Bus Assignment/103
  Constant108/1 -> Cast To Boolean2/1
  Constant69/1 -> Bus Assignment/69
  Bus Selector/53 -> Display57/1  "<meanVelocityZ>"
  Bus Selector/148 -> Display166/1  "<numTaskOverloads3>"
  Bus Selector/23 -> Display33/1  "<timestampUTC>"
  Constant58/1 -> Bus Assignment/58
  Constant50/1 -> Bus Assignment/50
  Constant17/1 -> Bus Assignment/16
  Constant152/1 -> Cast To Boolean18/1
  Bus Selector/45 -> Display39/1  "<velocityX>"
  Constant90/1 -> Bus Assignment/90
  Bus Selector/27 -> Display21/1  "<numSat>"
  Constant134/1 -> Bus Assignment/139
  Constant113/1 -> Bus Assignment/113
  Bus Selector/106 -> Display94/1  "<actuatorsEnabled>"
  Bus Selector/34 -> Display60/1  "<velocityX>"
  Constant150/1 -> Cast To Boolean11/1
  Constant89/1 -> Bus Assignment/89
  Constant145/1 -> Bus Assignment/151
  Bus Selector/42 -> Display36/1  "<meanVelocityZ>"
  Unpack MESSIN State Message/1 -> Display1/1
  Constant106/1 -> Cast To Boolean/1
  Bus Selector/95 -> Display82/1  "<torqeedoCurrent>"
  Bus Selector/127 -> Display110/1  "<velocityP>"
  Bus Selector/51 -> Display54/1  "<beamDistance3>"
  Bus Selector/1 -> Display2/1  "<timestampUTC>"
  Constant118/1 -> Cast To Boolean5/1
  Constant123/1 -> Bus Assignment/123
  Constant60/1 -> Bus Assignment/60
  Bus Selector/82 -> Display85/1  "<torqeedoTemperatureStator>"
  Bus Selector/109 -> Display97/1  "<externModeEnabled>"
  Constant115/1 -> Bus Assignment/115
  Bus Selector/150 -> Display177/1  "<numLostTicks>"
  Bus Selector/85 -> Display89/1  "<rudderServoSpeed>"
  Constant100/1 -> Bus Assignment/100
  Constant57/1 -> Bus Assignment/57
  Bus Selector/96 -> Display103/1  "<torqeedoTemperaturePCB>"
  Constant121/1 -> Bus Assignment/121
  Bus Selector/67 -> Display109/1  "<voltage>"
  Bus Selector/26 -> Display20/1  "<altitude>"
  Cast To Boolean5/1 -> Bus Assignment/118
  Constant88/1 -> Bus Assignment/88
  Bus Selector/114 -> Display113/1  "<positionLongitude>"
  Bus Selector/2 -> Display3/1  "<timestampUTC>"
  Constant32/1 -> Bus Assignment/27
  Constant46/1 -> Bus Assignment/46
  Bus Selector/8 -> Display9/1  "<velocityDown>"
  Bus Selector/35 -> Display61/1  "<velocityY>"
  Constant37/1 -> Bus Assignment/37
  Constant132/1 -> Bus Assignment/137
